simulink model "gradients"  (R2020b)
settings: Solver=VariableStepAuto  StartTime=0.0  StopTime=5  RelTol=1e-3
undefined symbols (not defined in the file): COLS, messi_blurred
libraries: visionhdlio x3
settings Model: Creator=Ethan  LastModifiedBy=Ethan
settings DebuggingCC: SignalRangeChecking=warning

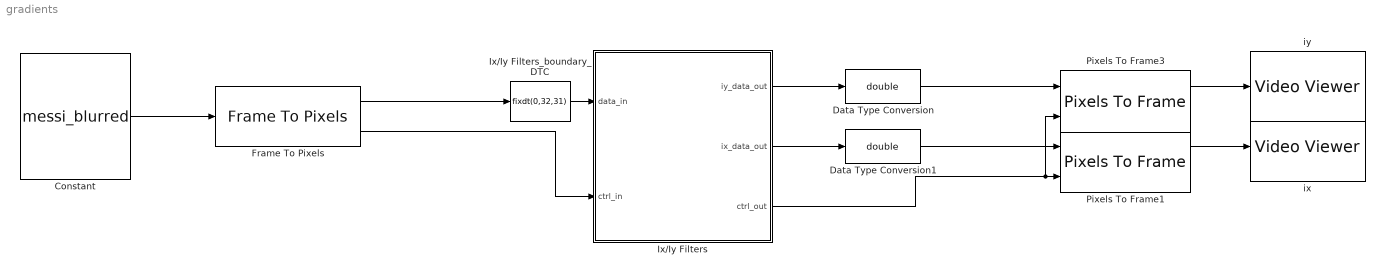
== system gradients ==
  Constant : Constant  Value=messi_blurred  OutDataTypeStr=double  SampleTime=1
  Data Type Conversion : DataTypeConversion  OutDataTypeStr=double
  Data Type Conversion1 : DataTypeConversion  OutDataTypeStr=double
  Frame To Pixels : visionhdlio/Frame To Pixels  NumComponents=1  NumPixels=1  VideoFormat=Custom  ActivePixelsPerLine=752  ActiveVideoLines=480  TotalPixelsPerLine=752  TotalVideoLines=480  StartingActiveLine=1  FrontPorch=0  SampleTime=0
      settings: SourceProductBaseCode=VT
  Ix/Iy Filters : Subsystem
  Ix/Iy Filters_boundary_DTC : DataTypeConversion  OutDataTypeStr=fixdt(0,32,31)  SaturateOnIntegerOverflow=on  RndMeth=Zero
  Pixels To Frame1 : visionhdlio/Pixels To Frame  NumComponents=1  NumPixels=1  VideoFormat=Custom  ActivePixelsPerLine=752  ActiveVideoLines=480  TotalPixelsPerLine=752  TotalVideoLines=480
      settings: SourceProductBaseCode=VT
  Pixels To Frame3 : visionhdlio/Pixels To Frame  NumComponents=1  NumPixels=1  VideoFormat=Custom  ActivePixelsPerLine=752  ActiveVideoLines=480  TotalPixelsPerLine=752  TotalVideoLines=480
      settings: SourceProductBaseCode=VT
  ix : VideoViewer  FigPos=[64 1077 927 969]
  iy : VideoViewer  FigPos=[993 1077 927 969]
  wires:
  Frame To Pixels/2 -> Ix/Iy Filters/2(ctrl_in)
  Pixels To Frame3/1 -> iy/1
  Ix/Iy Filters/1(iy_data_out) -> Data Type Conversion/1
  Data Type Conversion/1 -> Pixels To Frame3/1
  Pixels To Frame1/1 -> ix/1
  Data Type Conversion1/1 -> Pixels To Frame1/1
  Ix/Iy Filters/2(ix_data_out) -> Data Type Conversion1/1
  Ix/Iy Filters/3(ctrl_out) -> Pixels To Frame3/2, Pixels To Frame1/2
  Constant/1 -> Frame To Pixels/1
  Frame To Pixels/1 -> Ix/Iy Filters_boundary_DTC/1
  Ix/Iy Filters_boundary_DTC/1 -> Ix/Iy Filters/1(data_in)

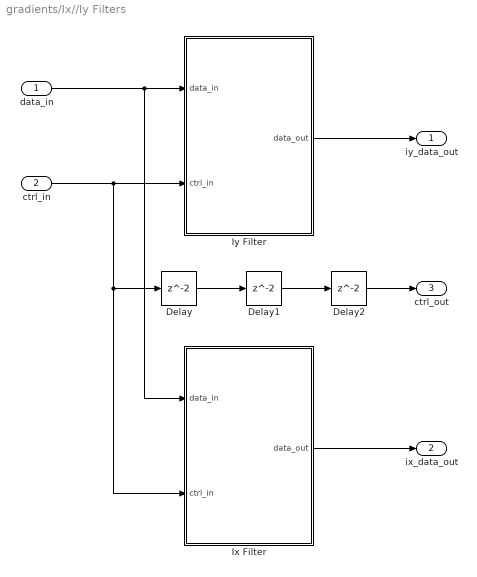
== system gradients/Ix//Iy Filters ==
  data_in : Inport
  ctrl_in : Inport  Port=2
  Delay : Delay
  Delay1 : Delay
  Delay2 : Delay
  Ix Filter : Subsystem
  Iy Filter : Subsystem
  iy_data_out : Outport
  ix_data_out : Outport  Port=2
  ctrl_out : Outport  Port=3
  wires:
  ctrl_in/1 -> Iy Filter/2(ctrl_in), Ix Filter/2(ctrl_in), Delay/1
  Iy Filter/1(data_out) -> iy_data_out/1
  data_in/1 -> Iy Filter/1(data_in), Ix Filter/1(data_in)
  Delay2/1 -> ctrl_out/1
  Delay1/1 -> Delay2/1
  Delay/1 -> Delay1/1
  Ix Filter/1(data_out) -> ix_data_out/1

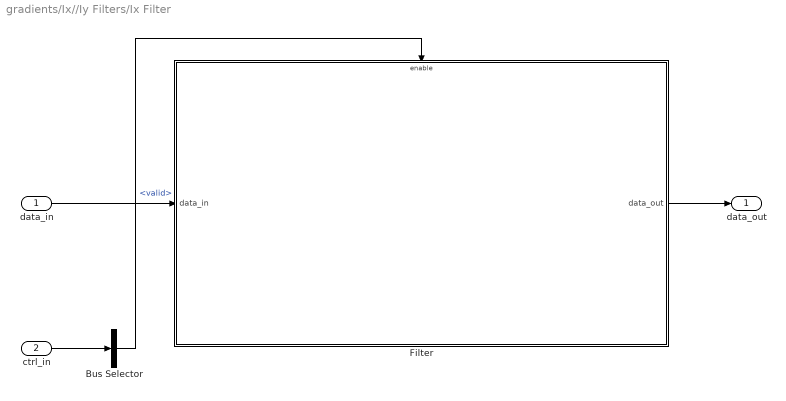
== system gradients/Ix//Iy Filters/Ix Filter ==
  data_in : Inport
  ctrl_in : Inport  Port=2
  Bus Selector : BusSelector  OutputSignals=valid
  Filter : Subsystem
  data_out : Outport
  wires:
  ctrl_in/1 -> Bus Selector/1
  data_in/1 -> Filter/1(data_in)
  Filter/1(data_out) -> data_out/1
  Bus Selector/1 -> Filter/Enable  "<valid>"

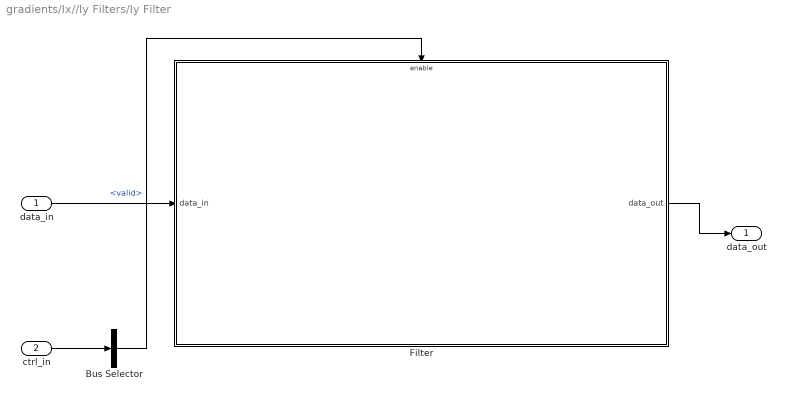
== system gradients/Ix//Iy Filters/Iy Filter ==
  data_in : Inport
  ctrl_in : Inport  Port=2
  Bus Selector : BusSelector  OutputSignals=valid
  Filter : Subsystem
  data_out : Outport
  wires:
  ctrl_in/1 -> Bus Selector/1
  data_in/1 -> Filter/1(data_in)
  Filter/1(data_out) -> data_out/1
  Bus Selector/1 -> Filter/Enable  "<valid>"

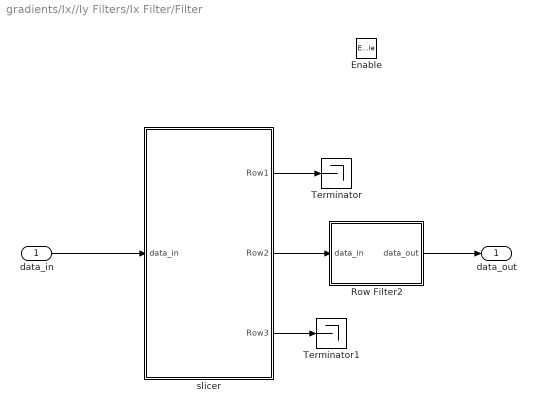
== system gradients/Ix//Iy Filters/Ix Filter/Filter ==
  data_in : Inport
  Enable : EnablePort
  Row Filter2 : Subsystem
  Terminator : Terminator
  Terminator1 : Terminator
  slicer : Subsystem
  data_out : Outport
  wires:
  data_in/1 -> slicer/1(data_in)
  slicer/2(Row2) -> Row Filter2/1(data_in)
  Row Filter2/1(data_out) -> data_out/1
  slicer/1(Row1) -> Terminator/1
  slicer/3(Row3) -> Terminator1/1

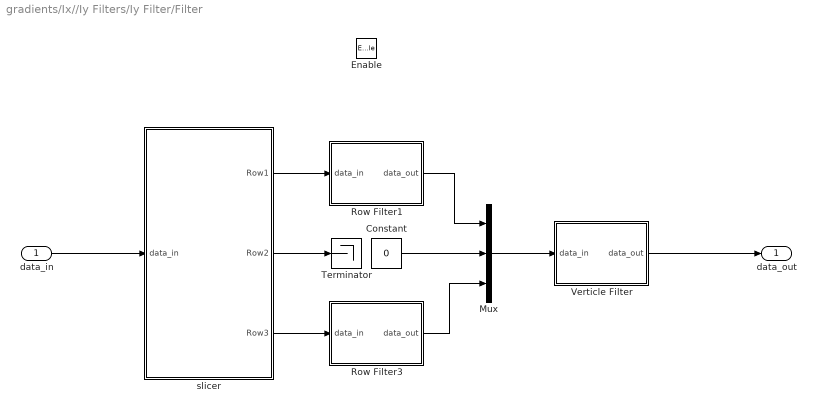
== system gradients/Ix//Iy Filters/Iy Filter/Filter ==
  data_in : Inport
  Enable : EnablePort
  Constant : Constant  Value=0  OutDataTypeStr=Inherit: Inherit via back propagation  SampleTime=-1
  Mux : Mux  Inputs=3
  Row Filter1 : Subsystem
  Row Filter3 : Subsystem
  Terminator : Terminator
  Verticle Filter : Subsystem
  slicer : Subsystem
  data_out : Outport
  wires:
  Row Filter1/1(data_out) -> Mux/1
  slicer/1(Row1) -> Row Filter1/1(data_in)
  data_in/1 -> slicer/1(data_in)
  slicer/2(Row2) -> Terminator/1
  slicer/3(Row3) -> Row Filter3/1(data_in)
  Mux/1 -> Verticle Filter/1(data_in)
  Verticle Filter/1(data_out) -> data_out/1
  Row Filter3/1(data_out) -> Mux/3
  Constant/1 -> Mux/2

== system gradients/Ix//Iy Filters/Ix Filter/Filter/Row Filter2 ==
  data_in : Inport
  Delay : Delay  DelayLength=4
  Symmetry : Subsystem
  data_out : Outport
  wires:
  Symmetry/1(data_out) -> Delay/1
  data_in/1 -> Symmetry/1(data_in)
  Delay/1 -> data_out/1

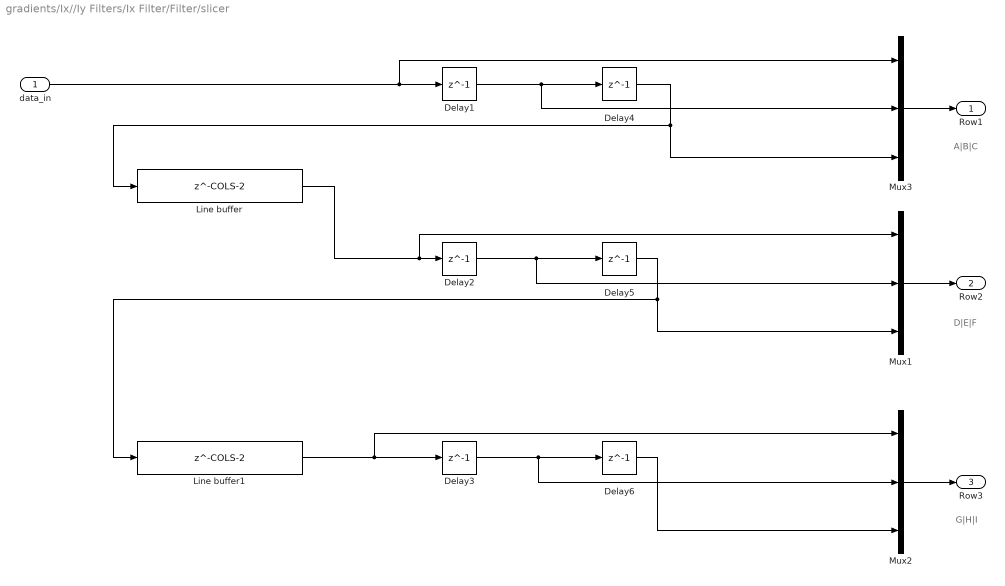
== system gradients/Ix//Iy Filters/Ix Filter/Filter/slicer ==
  note: A|B|C
  note: D|E|F
  note: G|H|I
  data_in : Inport
  Delay{1..6} (6 alike) : Delay  DelayLength=1  InitialCondition=0
  Line buffer : Delay  DelayLength=COLS-2  InitialCondition=0
  Line buffer1 : Delay  DelayLength=COLS-2  InitialCondition=0
  Mux1 : Mux  Inputs=3
  Mux2 : Mux  Inputs=3
  Mux3 : Mux  Inputs=3
  Row1 : Outport  VectorParamsAs1DForOutWhenUnconnected=off
  Row2 : Outport  Port=2  VectorParamsAs1DForOutWhenUnconnected=off
  Row3 : Outport  Port=3  VectorParamsAs1DForOutWhenUnconnected=off
  wires:
  Delay4/1 -> Mux3/3, Line buffer/1
  data_in/1 -> Mux3/1, Delay1/1
  Delay1/1 -> Mux3/2, Delay4/1
  Delay3/1 -> Mux2/2, Delay6/1
  Delay5/1 -> Mux1/3, Line buffer1/1
  Delay6/1 -> Mux2/3
  Line buffer/1 -> Mux1/1, Delay2/1
  Line buffer1/1 -> Mux2/1, Delay3/1
  Delay2/1 -> Mux1/2, Delay5/1
  Mux1/1 -> Row2/1
  Mux2/1 -> Row3/1
  Mux3/1 -> Row1/1

== system gradients/Ix//Iy Filters/Iy Filter/Filter/Row Filter1 ==
  data_in : Inport
  Delay : Delay
  Symmetry : Subsystem
  data_out : Outport
  wires:
  Symmetry/1(data_out) -> Delay/1
  data_in/1 -> Symmetry/1(data_in)
  Delay/1 -> data_out/1

== system gradients/Ix//Iy Filters/Iy Filter/Filter/Row Filter3 ==
  data_in : Inport
  Delay : Delay
  Symmetry : Subsystem
  data_out : Outport
  wires:
  Symmetry/1(data_out) -> Delay/1
  data_in/1 -> Symmetry/1(data_in)
  Delay/1 -> data_out/1

== system gradients/Ix//Iy Filters/Iy Filter/Filter/Verticle Filter ==
  data_in : Inport
  Delay2 : Delay
  Symmetry : Subsystem
  data_out : Outport
  wires:
  Delay2/1 -> data_out/1
  data_in/1 -> Symmetry/1(data_in)
  Symmetry/1(data_out) -> Delay2/1

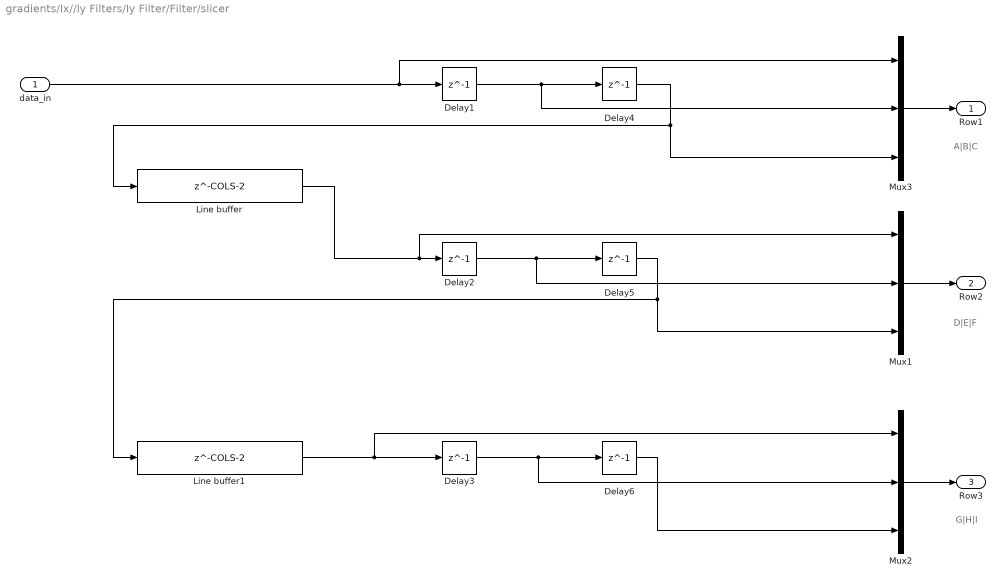
== system gradients/Ix//Iy Filters/Iy Filter/Filter/slicer ==
  note: A|B|C
  note: D|E|F
  note: G|H|I
  data_in : Inport
  Delay{1..6} (6 alike) : Delay  DelayLength=1  InitialCondition=0
  Line buffer : Delay  DelayLength=COLS-2  InitialCondition=0
  Line buffer1 : Delay  DelayLength=COLS-2  InitialCondition=0
  Mux1 : Mux  Inputs=3
  Mux2 : Mux  Inputs=3
  Mux3 : Mux  Inputs=3
  Row1 : Outport  VectorParamsAs1DForOutWhenUnconnected=off
  Row2 : Outport  Port=2  VectorParamsAs1DForOutWhenUnconnected=off
  Row3 : Outport  Port=3  VectorParamsAs1DForOutWhenUnconnected=off
  wires:
  Delay4/1 -> Mux3/3, Line buffer/1
  data_in/1 -> Mux3/1, Delay1/1
  Delay1/1 -> Mux3/2, Delay4/1
  Delay3/1 -> Mux2/2, Delay6/1
  Delay5/1 -> Mux1/3, Line buffer1/1
  Delay6/1 -> Mux2/3
  Line buffer/1 -> Mux1/1, Delay2/1
  Line buffer1/1 -> Mux2/1, Delay3/1
  Delay2/1 -> Mux1/2, Delay5/1
  Mux1/1 -> Row2/1
  Mux2/1 -> Row3/1
  Mux3/1 -> Row1/1

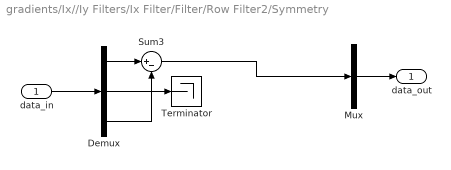
== system gradients/Ix//Iy Filters/Ix Filter/Filter/Row Filter2/Symmetry ==
  data_in : Inport
  Demux : Demux  Outputs=3
  Mux : Mux  Inputs=1
  Sum3 : Sum  Inputs=|+-  AccumDataTypeStr=fixdt(1,32,30)  OutDataTypeStr=fixdt(1,32,30)
  Terminator : Terminator
  data_out : Outport
  wires:
  Sum3/1 -> Mux/1
  data_in/1 -> Demux/1
  Demux/2 -> Terminator/1
  Demux/3 -> Sum3/2
  Demux/1 -> Sum3/1
  Mux/1 -> data_out/1

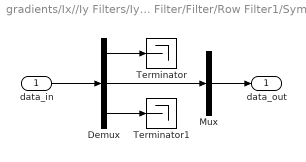
== system gradients/Ix//Iy Filters/Iy Filter/Filter/Row Filter1/Symmetry ==
  data_in : Inport
  Demux : Demux  Outputs=3
  Mux : Mux  Inputs=1
  Terminator : Terminator
  Terminator1 : Terminator
  data_out : Outport
  wires:
  data_in/1 -> Demux/1
  Demux/2 -> Mux/1
  Mux/1 -> data_out/1
  Demux/1 -> Terminator/1
  Demux/3 -> Terminator1/1

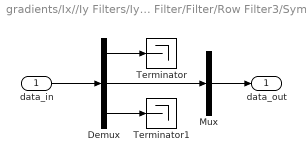
== system gradients/Ix//Iy Filters/Iy Filter/Filter/Row Filter3/Symmetry ==
  data_in : Inport
  Demux : Demux  Outputs=3
  Mux : Mux  Inputs=1
  Terminator : Terminator
  Terminator1 : Terminator
  data_out : Outport
  wires:
  data_in/1 -> Demux/1
  Demux/2 -> Mux/1
  Mux/1 -> data_out/1
  Demux/1 -> Terminator/1
  Demux/3 -> Terminator1/1

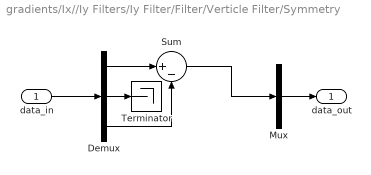
== system gradients/Ix//Iy Filters/Iy Filter/Filter/Verticle Filter/Symmetry ==
  data_in : Inport
  Demux : Demux  Outputs=3
  Mux : Mux  Inputs=1
  Sum : Sum  Inputs=|+-  AccumDataTypeStr=fixdt(1,32,30)  OutDataTypeStr=fixdt(1,32,30)
  Terminator : Terminator
  data_out : Outport
  wires:
  data_in/1 -> Demux/1
  Demux/2 -> Terminator/1
  Mux/1 -> data_out/1
  Demux/1 -> Sum/1
  Demux/3 -> Sum/2
  Sum/1 -> Mux/1
